simulink library "lib_rigid_body_dynamics"  (Simulink 8.8)
settings: Solver=ode45  StartTime=0.0  StopTime=10.0  RelTol=1e-3  EnableMultiTasking=on
values from neighbouring files (symbols this model uses):
  lambda = v    [inertia_nCRB_vp1_m.m]
undefined symbols (not defined in the file or in its folder): g_W, I, m, omega0_t0, r0, r2quat, r_B_B_C, R_t0, rD0
undefined symbols (not defined in the file): I_B_C, R_W_B_t0
libraries: lib_rigid_body_kinematics x9, lib_rigid_body_dynamics x4
settings Model: SuppressorTable=22 serialization::archive 11 0 3 0 0 0 11 0  Creator=schappler  LastModifiedBy=schappler

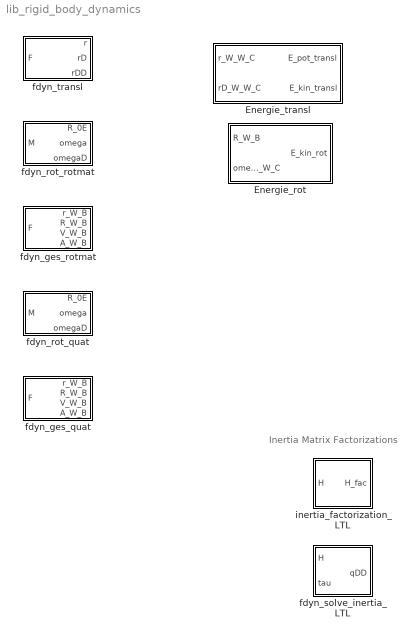
== system lib_rigid_body_dynamics ==
  note: Inertia Matrix Factorizations
  Energie_rot : Subsystem  mask{I_B_C=I_B_C}
      mask prompts: I_B_C "Traegheitstensor"
  Energie_transl : Subsystem  mask{m=m, g_W=g_W}
      mask prompts: m "Masse"; g_W "Gravitation"
  fdyn_ges_quat : Subsystem  mask{I=I_B_C, m=m, r0=r0, rD0=rD0, R_t0=R_W_B_t0, omega0_t0=omega0_t0, r_B_B_C=r_B_B_C}
      mask prompts: I "Trägheitstensor (3x3)"; m "Masse"; r0 "Anfangsposition"; rD0 "Anfangsgeschwindigkeit"; R_t0 "Anfangsrotation (3x3)"; omega0_t0 "Anfangsdrehgeschwindigkeit (3x1)"; r_B_B_C "Schwerpunktskoordinaten"
  fdyn_ges_rotmat : Subsystem  mask{I=I_B_C, m=m, r0=r0, rD0=rD0, R_t0=R_W_B_t0, omega0_t0=omega0_t0, r_B_B_C=r_B_B_C}
      mask prompts: I "Trägheitstensor (3x3)"; m "Masse"; r0 "Anfangsposition"; rD0 "Anfangsgeschwindigkeit"; R_t0 "Anfangsrotation (3x3)"; omega0_t0 "Anfangsdrehgeschwindigkeit (3x1)"; r_B_B_C "Schwerpunktskoordinaten"
  fdyn_rot_quat : Subsystem  mask{I=I, R_0E_t0=R_t0, omega0_t0=omega0_t0}
      mask prompts: I "Trägheitstensor (3x3)"; R_0E_t0 "Anfangsrotation (3x3)"; omega0_t0 "Anfangsdrehgeschwindigkeit (3x1)"
  fdyn_rot_rotmat : Subsystem  mask{I=I, R_0E_t0=R_t0, omega0_t0=omega0_t0}
      mask prompts: I "Trägheitstensor (3x3)"; R_0E_t0 "Anfangsrotation (3x3)"; omega0_t0 "Anfangsdrehgeschwindigkeit (3x1)"
  fdyn_solve_inertia_LTL : Subsystem  mask{lambda=lambda}
      mask prompts: lambda "Vorgänger-Indizes (lambda)"
      mask help:
      | Lösung des Gleichungssystems der Vorwärtsdynamik H*qDD=tau nach Featherstone2008.
      | Eingang ist die zerlegte Massenmatrix mit der LTL-Methode.
  fdyn_transl : Subsystem  mask{m=m, r0=r0, rD0=rD0}
      mask prompts: m "Masse (1x1)"; r0 "Anfangsposition (3x1)"; rD0 "Anfangsgeschwindigkeit (3x1)"
  inertia_factorization_LTL : Subsystem  mask{lambda=lambda}
      mask prompts: lambda "Vorgänger-Indizes (lambda)"
      mask help: Zerlegung der Massenmatrix eines Mehrkörpersystems nach Featherstone2008.
      mask DialogControl Control2 Prompt: Siehe Featherstone 2008

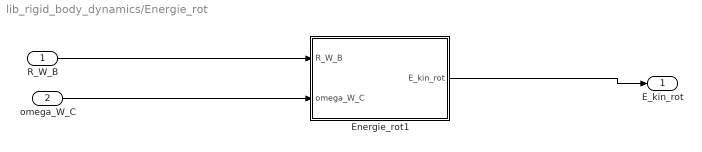
== system lib_rigid_body_dynamics/Energie_rot ==
  R_W_B : Inport
  omega_W_C : Inport  Port=2
  Energie_rot1 : MATLAB Function  TreatAsAtomicUnit=on
  E_kin_rot : Outport
  wires:
  R_W_B/1 -> Energie_rot1/1(R_W_B)
  omega_W_C/1 -> Energie_rot1/2(omega_W_C)
  Energie_rot1/1(E_kin_rot) -> E_kin_rot/1

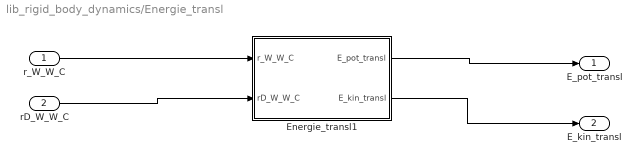
== system lib_rigid_body_dynamics/Energie_transl ==
  r_W_W_C : Inport
  rD_W_W_C : Inport  Port=2
  Energie_transl1 : MATLAB Function  TreatAsAtomicUnit=on
  E_pot_transl : Outport
  E_kin_transl : Outport  Port=2
  wires:
  rD_W_W_C/1 -> Energie_transl1/2(rD_W_W_C)
  r_W_W_C/1 -> Energie_transl1/1(r_W_W_C)
  Energie_transl1/1(E_pot_transl) -> E_pot_transl/1
  Energie_transl1/2(E_kin_transl) -> E_kin_transl/1

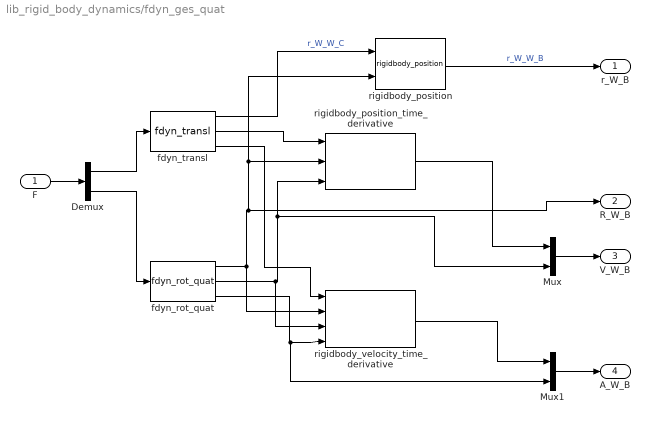
== system lib_rigid_body_dynamics/fdyn_ges_quat ==
  F : Inport  PortDimensions=6
  Demux : Demux  Outputs=[3 3]
  Mux : Mux  Inputs=2
  Mux1 : Mux  Inputs=2
  fdyn_rot_quat : lib_rigid_body_dynamics/fdyn_rot_quat  I=I  R_0E_t0=R_t0  omega0_t0=omega0_t0
  fdyn_transl : lib_rigid_body_dynamics/fdyn_transl  m=m  r0=r0+R_t0*r_B_B_C  rD0=rD0+cross(omega0_t0, R_t0*r_B_B_C)
  rigidbody_position : lib_rigid_body_kinematics/rigidbody_position  r_B_B_C=-r_B_B_C  PktName_B='C'  PktName_C='B'
  rigidbody_position_time_derivative : lib_rigid_body_kinematics/rigidbody_position_time_derivative  r_B_B_C=-r_B_B_C  PktName_B='C'  PktName_C='B'
  rigidbody_velocity_time_derivative : lib_rigid_body_kinematics/rigidbody_velocity_time_derivative  r_B_B_C=-r_B_B_C  PktName_B='C'  PktName_C='B'
  r_W_B : Outport  PortDimensions=3
  R_W_B : Outport  Port=2  PortDimensions=[3 3]
  V_W_B : Outport  Port=3  PortDimensions=6
  A_W_B : Outport  Port=4  PortDimensions=6
  wires:
  Mux/1 -> V_W_B/1
  Mux1/1 -> A_W_B/1
  fdyn_rot_quat/3 -> rigidbody_velocity_time_derivative/4, Mux1/2
  fdyn_rot_quat/2 -> rigidbody_velocity_time_derivative/3, rigidbody_position_time_derivative/3, Mux/2
  fdyn_rot_quat/1 -> rigidbody_velocity_time_derivative/2, rigidbody_position_time_derivative/2, rigidbody_position/2, R_W_B/1
  fdyn_transl/1 -> rigidbody_position/1  "r_W_W_C"
  F/1 -> Demux/1
  Demux/1 -> fdyn_transl/1
  Demux/2 -> fdyn_rot_quat/1
  fdyn_transl/2 -> rigidbody_position_time_derivative/1
  rigidbody_position_time_derivative/1 -> Mux/1
  fdyn_transl/3 -> rigidbody_velocity_time_derivative/1
  rigidbody_velocity_time_derivative/1 -> Mux1/1
  rigidbody_position/1 -> r_W_B/1  "r_W_W_B"

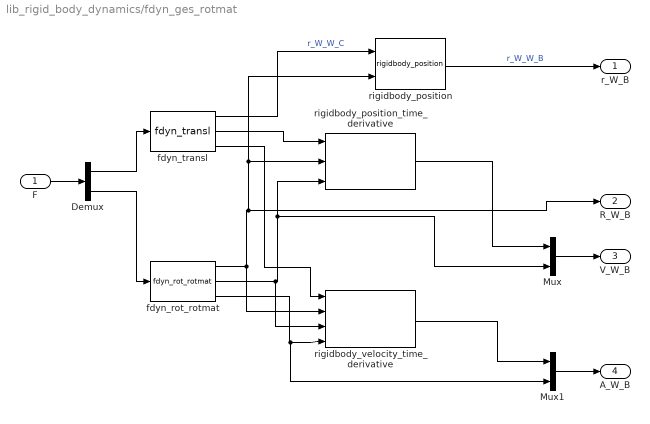
== system lib_rigid_body_dynamics/fdyn_ges_rotmat ==
  F : Inport  PortDimensions=6
  Demux : Demux  Outputs=[3 3]
  Mux : Mux  Inputs=2
  Mux1 : Mux  Inputs=2
  fdyn_rot_rotmat : lib_rigid_body_dynamics/fdyn_rot_rotmat  I=I  R_0E_t0=R_t0  omega0_t0=omega0_t0
  fdyn_transl : lib_rigid_body_dynamics/fdyn_transl  m=m  r0=r0+R_t0*r_B_B_C  rD0=rD0+cross(omega0_t0, R_t0*r_B_B_C)
  rigidbody_position : lib_rigid_body_kinematics/rigidbody_position  r_B_B_C=-r_B_B_C  PktName_B='C'  PktName_C='B'
  rigidbody_position_time_derivative : lib_rigid_body_kinematics/rigidbody_position_time_derivative  r_B_B_C=-r_B_B_C  PktName_B='C'  PktName_C='B'
  rigidbody_velocity_time_derivative : lib_rigid_body_kinematics/rigidbody_velocity_time_derivative  r_B_B_C=-r_B_B_C  PktName_B='C'  PktName_C='B'
  r_W_B : Outport  PortDimensions=3
  R_W_B : Outport  Port=2  PortDimensions=[3 3]
  V_W_B : Outport  Port=3  PortDimensions=6
  A_W_B : Outport  Port=4  PortDimensions=6
  wires:
  Mux/1 -> V_W_B/1
  Mux1/1 -> A_W_B/1
  fdyn_rot_rotmat/3 -> rigidbody_velocity_time_derivative/4, Mux1/2
  fdyn_rot_rotmat/2 -> rigidbody_velocity_time_derivative/3, rigidbody_position_time_derivative/3, Mux/2
  fdyn_rot_rotmat/1 -> rigidbody_velocity_time_derivative/2, rigidbody_position_time_derivative/2, rigidbody_position/2, R_W_B/1
  fdyn_transl/1 -> rigidbody_position/1  "r_W_W_C"
  F/1 -> Demux/1
  Demux/1 -> fdyn_transl/1
  Demux/2 -> fdyn_rot_rotmat/1
  fdyn_transl/2 -> rigidbody_position_time_derivative/1
  rigidbody_position_time_derivative/1 -> Mux/1
  fdyn_transl/3 -> rigidbody_velocity_time_derivative/1
  rigidbody_velocity_time_derivative/1 -> Mux1/1
  rigidbody_position/1 -> r_W_B/1  "r_W_W_B"

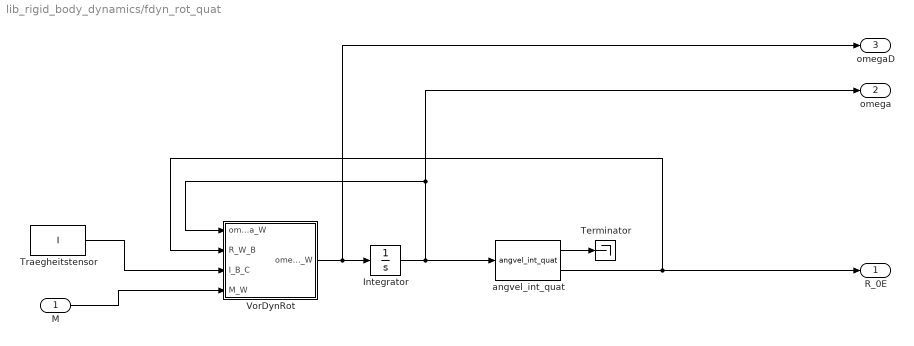
== system lib_rigid_body_dynamics/fdyn_rot_quat ==
  M : Inport  PortDimensions=3
  Integrator : Integrator  InitialCondition=omega0_t0
  Terminator : Terminator
  Traegheitstensor : Constant  Value=I
  VorDynRot : MATLAB Function  TreatAsAtomicUnit=on
  angvel_int_quat : lib_rigid_body_kinematics/angvel_int_quat  quat_t0=r2quat(R_t0)
  R_0E : Outport  PortDimensions=[3 3]
  omega : Outport  Port=2  PortDimensions=3
  omegaD : Outport  Port=3  PortDimensions=3
  wires:
  Traegheitstensor/1 -> VorDynRot/3(I_B_C)
  VorDynRot/1(omegaD_W) -> omegaD/1, Integrator/1
  Integrator/1 -> angvel_int_quat/1, VorDynRot/1(omega_W), omega/1
  angvel_int_quat/2 -> VorDynRot/2(R_W_B), R_0E/1
  M/1 -> VorDynRot/4(M_W)
  angvel_int_quat/1 -> Terminator/1

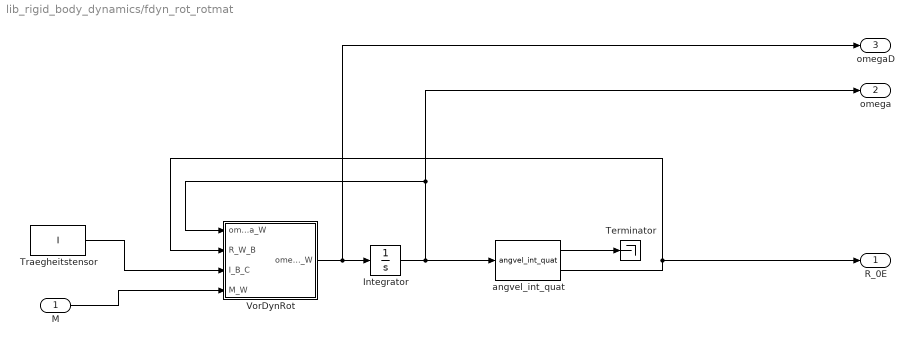
== system lib_rigid_body_dynamics/fdyn_rot_rotmat ==
  M : Inport  PortDimensions=3
  Integrator : Integrator  InitialCondition=omega0_t0
  Terminator : Terminator
  Traegheitstensor : Constant  Value=I
  VorDynRot : MATLAB Function  TreatAsAtomicUnit=on
  angvel_int_quat : lib_rigid_body_kinematics/angvel_int_quat  quat_t0=r2quat(R_0E_t0)  KSName_B='B'  KSName_W='W'
  R_0E : Outport  PortDimensions=[3 3]
  omega : Outport  Port=2  PortDimensions=3
  omegaD : Outport  Port=3  PortDimensions=3
  wires:
  Traegheitstensor/1 -> VorDynRot/3(I_B_C)
  VorDynRot/1(omegaD_W) -> omegaD/1, Integrator/1
  Integrator/1 -> VorDynRot/1(omega_W), omega/1, angvel_int_quat/1
  angvel_int_quat/2 -> VorDynRot/2(R_W_B), R_0E/1
  M/1 -> VorDynRot/4(M_W)
  angvel_int_quat/1 -> Terminator/1

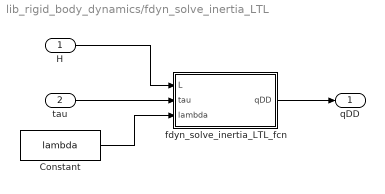
== system lib_rigid_body_dynamics/fdyn_solve_inertia_LTL ==
  H : Inport
  tau : Inport  Port=2
  Constant : Constant  Value=lambda
  fdyn_solve_inertia_LTL_fcn : MATLAB Function  TreatAsAtomicUnit=on
  qDD : Outport
  wires:
  H/1 -> fdyn_solve_inertia_LTL_fcn/1(L)
  fdyn_solve_inertia_LTL_fcn/1(qDD) -> qDD/1
  Constant/1 -> fdyn_solve_inertia_LTL_fcn/3(lambda)
  tau/1 -> fdyn_solve_inertia_LTL_fcn/2(tau)

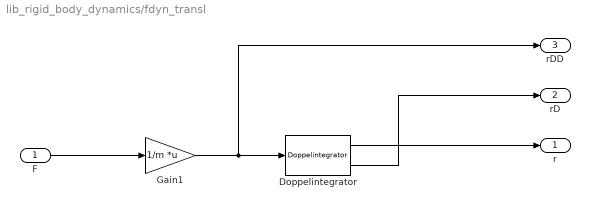
== system lib_rigid_body_dynamics/fdyn_transl ==
  F : Inport  PortDimensions=3
  Doppelintegrator : lib_rigid_body_kinematics/Doppelintegrator  r0=r0  rD0=rD0  Name_v='x'
  Gain1 : Gain  Gain=1/m  Multiplication=Matrix(K*u)
  r : Outport  PortDimensions=3
  rD : Outport  Port=2  PortDimensions=3
  rDD : Outport  Port=3  PortDimensions=3
  wires:
  Gain1/1 -> Doppelintegrator/1, rDD/1
  Doppelintegrator/1 -> r/1
  F/1 -> Gain1/1
  Doppelintegrator/2 -> rD/1

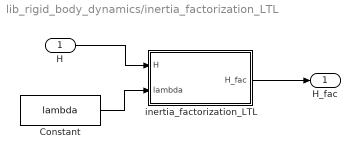
== system lib_rigid_body_dynamics/inertia_factorization_LTL ==
  H : Inport
  Constant : Constant  Value=lambda
  inertia_factorization_LTL : MATLAB Function  TreatAsAtomicUnit=on
  H_fac : Outport
  wires:
  H/1 -> inertia_factorization_LTL/1(H)
  inertia_factorization_LTL/1(H_fac) -> H_fac/1
  Constant/1 -> inertia_factorization_LTL/2(lambda)

== matlab function Energie_transl/Energie_transl1 ==
  data: r_W_W_C input double; E_pot_transl output double; m parameter double; E_kin_transl output double; rD_W_W_C input double; g_W parameter double
function [E_pot_transl, E_kin_transl] = fcn(r_W_W_C, m, rD_W_W_C, g_W)
%#codegen

assert(isa(r_W_W_C,'double') && isreal(r_W_W_C) && all(size(r_W_W_C) == [3 1]), ...
  'Position muss [3x1] double sein');

assert(isa(m,'double') && isreal(m) && all(size(m) == [1 1]), ...
  'Masse muss [1x1] double sein');

assert(isa(rD_W_W_C,'double') && isreal(rD_W_W_C) && all(size(rD_W_W_C) == [3 1]), ...
  'Geschwindigkeit muss [3x1] double sein');

E_pot_transl = -m * g_W' * r_W_W_C;

E_kin_transl = 0.5 * m * (rD_W_W_C' * rD_W_W_C);

== matlab function fdyn_rot_rotmat/VorDynRot ==
  data: omega_W input double; omegaD_W output double; R_W_B input double; I_B_C input double; M_W input double
% Quellen:
% [1] Robotik I Skript

function omegaD_W = euler(omega_W, R_W_B, I_B_C, M_W)
%% Init
%#codegen
assert(isa(omega_W,'double') && isreal(omega_W) && all(size(omega_W) == [3 1]), ...
  'Drehgeschwindigkeit muss [3x1] double sein.');
assert(isa(R_W_B,'double') && isreal(R_W_B) && all(size(R_W_B) == [3 3]), ...
  'Rotationsmatrix muss [3x3] double sein.');
assert(isa(I_B_C,'double') && isreal(I_B_C) && all(size(I_B_C) == [3 3]), ...
  'Traeghteitstensor muss [3x3] double sein.');
assert(isa(M_W,'double') && isreal(M_W) && all(size(M_W) == [3 1]), ...
  'Beschleunigungsmoment muss [3x1] double sein.');

%% Berechnung
% Trägheitstensor in Weltkoordinaten rotieren
% [1], S. 119, Equ. (7.26)
I_W_C = R_W_B * I_B_C * R_W_B';

% Euler-Gleichung (Drallsatz) nach Beschleunigung umformen
omegaD_W = I_W_C \ (M_W - cross(omega_W, (I_W_C*omega_W)));

== matlab function Energie_rot/Energie_rot1 ==
  data: R_W_B input double; I_B_C parameter double; omega_W_C input double; E_kin_rot output double
function E_kin_rot  = fcn(R_W_B, I_B_C, omega_W_C)
%#codegen

assert(isa(R_W_B,'double') && isreal(R_W_B) && all(size(R_W_B) == [3 3]), ...
  'Rotationsmatrix muss [3x3] double sein');
assert(isa(I_B_C,'double') && isreal(I_B_C) && all(size(I_B_C) == [3 3]), ...
  'Traegheitstensor muss [3x3] double sein');
assert(isa(omega_W_C,'double') && isreal(omega_W_C) && all(size(omega_W_C) == [3 1]), ...
  'Winkelgeschwindigkeit muss [3x1] double sein');

I_W_C = R_W_B * I_B_C * R_W_B';
E_kin_rot = 0.5 * omega_W_C' * (I_W_C * omega_W_C);

== matlab function fdyn_rot_quat/VorDynRot ==
  data: omega_W input double; omegaD_W output double; R_W_B input double; I_B_C input double; M_W input double
% Quellen:
% [1] Robotik I Skript

function omegaD_W = euler(omega_W, R_W_B, I_B_C, M_W)
%% Init
%#codegen
assert(isa(omega_W,'double') && isreal(omega_W) && all(size(omega_W) == [3 1]), ...
  'Drehgeschwindigkeit muss [3x1] double sein.');
assert(isa(R_W_B,'double') && isreal(R_W_B) && all(size(R_W_B) == [3 3]), ...
  'Rotationsmatrix muss [3x3] double sein.');
assert(isa(I_B_C,'double') && isreal(I_B_C) && all(size(I_B_C) == [3 3]), ...
  'Traeghteitstensor muss [3x3] double sein.');
assert(isa(M_W,'double') && isreal(M_W) && all(size(M_W) == [3 1]), ...
  'Beschleunigungsmoment muss [3x1] double sein.');

%% Berechnung
% Trägheitstensor in Weltkoordinaten rotieren
% [1], S. 119, Equ. (7.26)
I_W_C = R_W_B * I_B_C * R_W_B';

% Euler-Gleichung (Drallsatz) nach Beschleunigung umformen
omegaD_W = I_W_C \ (M_W - cross(omega_W, (I_W_C*omega_W)));

== matlab function inertia_factorization_LTL/inertia_factorization_LTL ==
  data: H_fac output double; H input double; lambda input double
% Faktorisiere eine Massenmatrix mit der LTL-Zerlegung
% 
% Moritz Schappler, schappler@irt.uni-hannover.de, 2016-12
% (c) Institut für Regelungstechnik, Universität Hannover

function H_fac = fcn(H, lambda)
%#codegen

H_fac = inertia_factorization_LTL(H, lambda);

== matlab function fdyn_solve_inertia_LTL/fdyn_solve_inertia_LTL_fcn ==
  data: qDD output double; L input double; tau input double; lambda input double
% Berechne die Beschleunigung aus gegebenem Beschleunigungsmoment und einer
% LTL-zerlegten Massenmatrix
% 
% Moritz Schappler, schappler@irt.uni-hannover.de, 2016-12
% (c) Institut für Regelungstechnik, Universität Hannover

function qDD = fcn(L, tau, lambda)
%#codegen

qDD =  fdyn_solve_inertia_LTL(L, tau, lambda);
